simulink library "tanksensing_lib"  (R2019b)
settings: Solver=VariableStepAuto  StartTime=0.0  StopTime=10.0  RelTol=1e-3
libraries: simulink x3
settings Model: Creator=CentoPas  LastModifiedBy=CentoPas

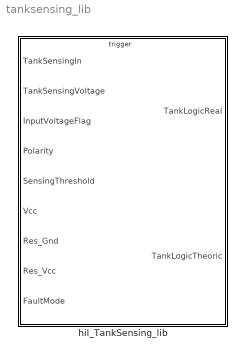
== system tanksensing_lib ==
  hil_TankSensing_lib : Subsystem  TreatAsAtomicUnit=on  RTWFcnName=hil_tanksensing_lib  mask(Tank Sensing){Parameter1={'TankSensingIn','single','0 - 1','Adim','Input sensing signal from tank'; 'TankSensingVoltage','single','0 - 5', 'V', 'Input voltage signal from tank';'InputVoltageFlag','uint8','0 - 1', 'Adim',' Flag to switch from adim input to voltage input';'Polarity','uint8','0 - 1','Adim','Command to invert polarity';'SensingThreshold','single','0 - max 32Bit','V','Comparing threshold for CMOS logic';'Vcc','single','0 - 5','V','Supply voltage';'Res_Gnd','single','0 - max 32Bit','Ohm','Pull-down resistance value';'Res_Vcc','single','0 - max 32Bit','Ohm','Pull-up resistance value';}, Parameter3={'FaultMode','uint8','0 - 2','Adim','Fault on sensing signal' }, Parameter2={'TankLogicReal','uint8','0 - 1','Adim','Output tank logic level after fault management';'TankLogicTheoric','uint8','0 - 1','Adim','Tank logic theoric level, no fault management'}}
      mask help:
      | The aim of this work is Model in Loop (MIL) testing of Tank Sensing. It is here studied the case of the circuit of the EDR16R schematic used for this purpose. The input signal can be a voltage signal or a logic signal that represents the tank fill level. In the second case, the input is multiplied by the Transfer Function value, which is calculated starting from the resistances values, thus becoming a voltage. Resistances are listed as tunable parameters and can simulate short circuits or open circuits.
      | Polarity and Fault management are also taken into account and can be simulated through their respective commands.
      | The output is a signal logic that expresses the emptyness or not of the tank.
      settings: RTWFcnNameOpts=User specified
      mask Help: https://sdlcwiki.electrolux.com/display/ASTMBDHIL/Tank+Sensing+@+EdmLib
      mask DialogControl Container5 Prompt: Inputs
      mask DialogControl Control2 Prompt: Failure Detection
      mask DialogControl Container7 Prompt: Outputs

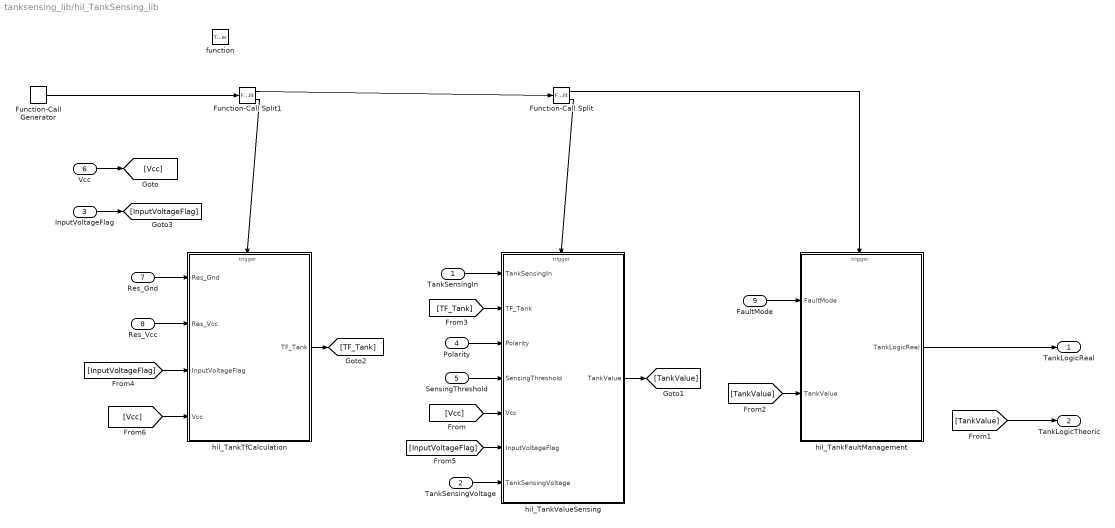
== system tanksensing_lib/hil_TankSensing_lib ==
  TankSensingIn : Inport  RequirementInfo={} %GIDa_b751ddf4_f7ab_455b_ad5f_57267e982822
  TankSensingVoltage : Inport  Port=2
  InputVoltageFlag : Inport  Port=3
  Polarity : Inport  Port=4
  "SensingThreshold " : Inport  Port=5
  Vcc : Inport  RequirementInfo={} %GIDa_577f5463_3c1c_4139_8bd3_238316ee9637  Port=6
  Res_Gnd : Inport  Port=7
  Res_Vcc : Inport  Port=8
  "FaultMode " : Inport  Port=9
  function : TriggerPort  TriggerType=function-call  VariantControl=Variant
  Function-Call Generator : simulink/Ports & Subsystems/Function-Call Generator  sample_time=-1  numberOfIterations=1
  Function-Call Split : FunctionCallSplit  NumOutputPorts=2  OutputPortLayout=default
  Function-Call Split1 : FunctionCallSplit  NumOutputPorts=2  OutputPortLayout=default
  hil_TankFaultManagement : Subsystem  TreatAsAtomicUnit=on
  hil_TankTfCalculation : Subsystem  TreatAsAtomicUnit=on
  hil_TankValueSensing : Subsystem  TreatAsAtomicUnit=on
  TankLogicReal : Outport  OutDataTypeStr=uint8
  TankLogicTheoric : Outport  Port=2  OutDataTypeStr=uint8
  wires:
  TankSensingIn/1 -> hil_TankValueSensing/1(TankSensingIn)
  Function-Call Split/2 -> hil_TankValueSensing/Trigger
  Vcc/1 -> [Vcc]
  Function-Call Split/1 -> hil_TankFaultManagement/Trigger
  hil_TankValueSensing/1("TankValue ") -> [TankValue]
  [TF_Tank] -> hil_TankValueSensing/2(TF_Tank)
  Polarity/1 -> hil_TankValueSensing/3(Polarity)
  "SensingThreshold "/1 -> hil_TankValueSensing/4(SensingThreshold)
  [Vcc] -> hil_TankValueSensing/5("Vcc ")
  [TankValue] -> hil_TankFaultManagement/2(TankValue)
  "FaultMode "/1 -> hil_TankFaultManagement/1(FaultMode)
  hil_TankFaultManagement/1(TankLogicReal) -> TankLogicReal/1
  [TankValue] -> TankLogicTheoric/1
  Function-Call Generator/1 -> Function-Call Split1/1
  Function-Call Split1/1 -> Function-Call Split/1
  Function-Call Split1/2 -> hil_TankTfCalculation/Trigger
  hil_TankTfCalculation/1(TF_Tank) -> [TF_Tank]
  Res_Gnd/1 -> hil_TankTfCalculation/1(Res_Gnd)
  Res_Vcc/1 -> hil_TankTfCalculation/2(Res_Vcc)
  InputVoltageFlag/1 -> [InputVoltageFlag]
  [InputVoltageFlag] -> hil_TankTfCalculation/3(InputVoltageFlag)
  [InputVoltageFlag] -> hil_TankValueSensing/6(InputVoltageFlag)
  TankSensingVoltage/1 -> hil_TankValueSensing/7(TankSensingVoltage)
  [Vcc] -> hil_TankTfCalculation/4("Vcc ")

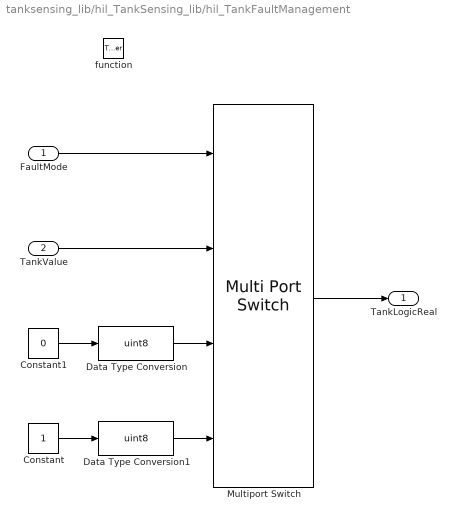
== system tanksensing_lib/hil_TankSensing_lib/hil_TankFaultManagement ==
  FaultMode : Inport
  TankValue : Inport  Port=2
  function : TriggerPort  TriggerType=function-call  VariantControl=Variant
  Constant : Constant
  Constant1 : Constant  Value=0
  Data Type Conversion : DataTypeConversion  OutDataTypeStr=uint8
  Data Type Conversion1 : DataTypeConversion  OutDataTypeStr=uint8
  Multiport Switch : MultiPortSwitch  DataPortOrder=Zero-based contiguous  DiagnosticForDefault=None  zeroidx=on
  TankLogicReal : Outport
  wires:
  Multiport Switch/1 -> TankLogicReal/1
  FaultMode/1 -> Multiport Switch/1
  TankValue/1 -> Multiport Switch/2
  Constant1/1 -> Data Type Conversion/1
  Constant/1 -> Data Type Conversion1/1
  Data Type Conversion/1 -> Multiport Switch/3
  Data Type Conversion1/1 -> Multiport Switch/4

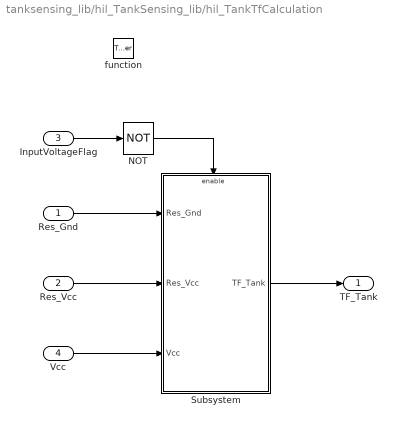
== system tanksensing_lib/hil_TankSensing_lib/hil_TankTfCalculation ==
  Res_Gnd : Inport
  Res_Vcc : Inport  Port=2
  InputVoltageFlag : Inport  Port=3
  "Vcc " : Inport  Port=4
  function : TriggerPort  TriggerType=function-call  VariantControl=Variant
  NOT : Logic  Operator=NOT  IconShape=distinctive  AllPortsSameDT=off  OutDataTypeStr=boolean
  Subsystem : Subsystem
  TF_Tank : Outport  OutDataTypeStr=single
  wires:
  Res_Gnd/1 -> Subsystem/1(Res_Gnd)
  Res_Vcc/1 -> Subsystem/2(Res_Vcc)
  Subsystem/1(TF_Tank) -> TF_Tank/1
  InputVoltageFlag/1 -> NOT/1
  NOT/1 -> Subsystem/Enable
  "Vcc "/1 -> Subsystem/3(Vcc)

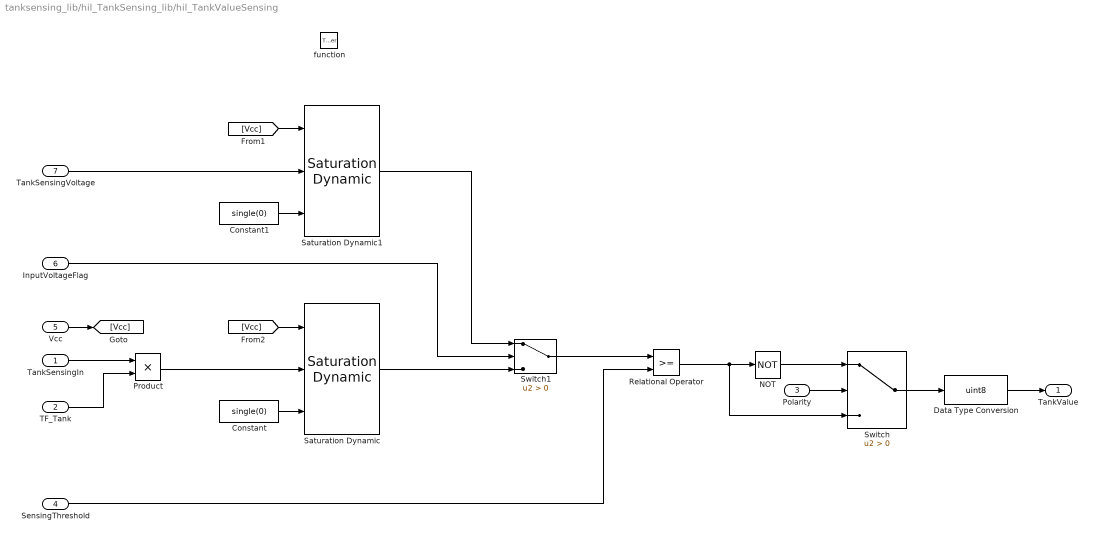
== system tanksensing_lib/hil_TankSensing_lib/hil_TankValueSensing ==
  TankSensingIn : Inport
  TF_Tank : Inport  Port=2
  Polarity : Inport  Port=3
  SensingThreshold : Inport  Port=4
  "Vcc " : Inport  Port=5
  InputVoltageFlag : Inport  Port=6
  TankSensingVoltage : Inport  Port=7
  function : TriggerPort  TriggerType=function-call  VariantControl=Variant
  Constant : Constant  Value=single(0)
  Constant1 : Constant  Value=single(0)
  Data Type Conversion : DataTypeConversion  OutDataTypeStr=uint8
  NOT : Logic  Operator=NOT  IconShape=distinctive  AllPortsSameDT=off  OutDataTypeStr=boolean
  Product : Product
  Relational Operator : RelationalOperator  OutDataTypeStr=boolean  RndMeth=Zero
  Saturation Dynamic : simulink/Discontinuities/Saturation Dynamic  OutMin=[]  OutMax=[]  OutDataTypeStr=Inherit: Same as second input  OutDataType=fixdt(1, 16)  OutScaling=2^-10  DoSatur=off
  Saturation Dynamic1 : simulink/Discontinuities/Saturation Dynamic  OutMin=[]  OutMax=[]  OutDataTypeStr=Inherit: Same as second input  OutDataType=fixdt(1, 16)  OutScaling=2^-10  DoSatur=off
  Switch : Switch  Criteria=u2 > Threshold
  Switch1 : Switch  Criteria=u2 > Threshold
  "TankValue " : Outport
  wires:
  TF_Tank/1 -> Product/2
  SensingThreshold/1 -> Relational Operator/2
  TankSensingIn/1 -> Product/1
  Polarity/1 -> Switch/2
  Switch/1 -> Data Type Conversion/1
  NOT/1 -> Switch/1
  Constant/1 -> Saturation Dynamic/3
  Relational Operator/1 -> Switch/3, NOT/1
  Data Type Conversion/1 -> "TankValue "/1
  Product/1 -> Saturation Dynamic/2
  Switch1/1 -> Relational Operator/1
  InputVoltageFlag/1 -> Switch1/2
  Saturation Dynamic/1 -> Switch1/3
  TankSensingVoltage/1 -> Saturation Dynamic1/2
  Saturation Dynamic1/1 -> Switch1/1
  Constant1/1 -> Saturation Dynamic1/3
  "Vcc "/1 -> [Vcc]
  [Vcc] -> Saturation Dynamic1/1
  [Vcc] -> Saturation Dynamic/1

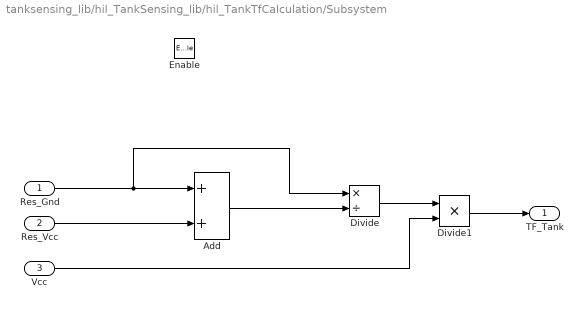
== system tanksensing_lib/hil_TankSensing_lib/hil_TankTfCalculation/Subsystem ==
  Res_Gnd : Inport
  Res_Vcc : Inport  Port=2
  Vcc : Inport  Port=3
  Enable : EnablePort
  Add : Sum
  Divide : Product  Inputs=*/
  Divide1 : Product  Inputs=**
  TF_Tank : Outport  OutDataTypeStr=single  OutputWhenDisabled=reset  InitialOutput=[single(0)]
  wires:
  Add/1 -> Divide/2
  Res_Vcc/1 -> Add/2
  Res_Gnd/1 -> Divide/1, Add/1
  Divide/1 -> Divide1/1
  Divide1/1 -> TF_Tank/1
  Vcc/1 -> Divide1/2
